simulink model "Ejemplo_5_1"  (R2013a)
settings: Solver=ode45  StartTime=0.0  StopTime=100  RelTol=1e-3
settings Model: Creator=Miguel  LastModifiedBy=Miguel

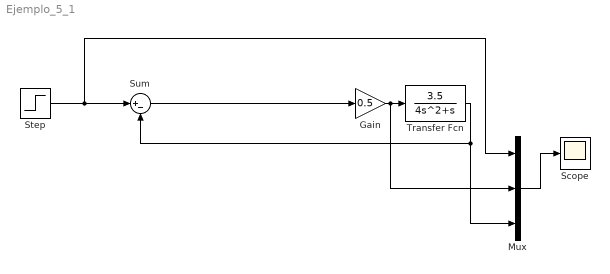
== system Ejemplo_5_1 ==
  Gain : Gain  Gain=0.5
  Mux : Mux  Inputs=3
  Scope : Scope
      settings: TickLabels=on  ShowLegends=on
  Step : Step  SampleTime=0
  Sum : Sum  Inputs=|+-
  Transfer Fcn : TransferFcn  Numerator=[3.5]  Denominator=[4 1 0]
  wires:
  Transfer Fcn/1 -> Mux/3, Sum/2
  Mux/1 -> Scope/1
  Step/1 -> Sum/1, Mux/1
  Gain/1 -> Mux/2, Transfer Fcn/1
  Sum/1 -> Gain/1
